simulink model "Compression_Gain_Calc"  (R2019a)
settings: Solver=FixedStepDiscrete  StartTime=0.0  StopTime=t_end  RelTol=1e-3
InitFcn:
  | clear;
  | DIAGNOSTIC = 0;  %% flag to give more information as simulation proceeds such as comments & plots
  | CALIB_DIAGNOSTIC =  0; %% flag to give more information about calibration of filterbank due to overlap between filters: Mar 2016
  | PRESCRIPT = 1;  %% flag to plot requested versus achieved insertion gains (esp for 125-250 Hz region).
  | ipfiledigrms = -36; %% input file RMS in dB for 65 dB SPL equivalent
  | opfiledigrms = -36; %% output file RMS in dB for 65 dB SPL equivalent
  | equiv_ipSPL = 65; %% simulation of signal at this level through aid`
  | X_high = 1; % Maximum input
  | ref_dB = 85; X_ref = 1; % Define a reference point in X and its dBA value
  | re_level = 10.^(.05*(equiv_ipSPL-65)); %% scale factor at start of hearing aid, to get input to desired simulation level
  | M_bits = 5;   % decides length of tables, 2^(4+M_bits)
  | 
  | NChans = 5;
  | [chan_cfs, chan_thrs, t_atts, t_rels] ...
  |    = InitializeCompressionSettings(NChans);
  | % AidSettings5Chans;
  | 
  | %[VALID_WAV_FILE, sig, Fs, nbits, file_rms_dB, NStreams] ...
  | %  = loadwavfile(ipfiledigrms); %%  find [Fs], performs [recalculate] externally, provided valid file found
  | VALID_WAV_FILE = 1;
  | %[newfile, newpath] = uigetfile('*.wav','Open Signal File To Process.....');
  | %if isequal(newfile,0) || isequal(newpath,0)
  | %    fprintf(1,'\nFile not found'); VALID_WAV_FILE = 0;
  | %else
  | %    [sig, Fs] = audioread(strcat(newpath,newfile));
  | %end
  | X_thresh = 1*10^(0.05*(0-85));
  | 
  | Amplitudes = [X_thresh, X_thresh*10, X_thresh*100, X_thresh*1000, X_thresh*10000, 1]; %, X_thresh*100000];
  | 
  | fMin = 100; %Hz
  | fMax = 10000; %Hz
  | Fs = 48000; %Hz
  | Ts = 1/Fs;
  | %tt = (0:length(sig)-1 )./Fs;
  | tt = 0:Ts:4;
  | deltaF = (fMax - fMin)/tt(end);
  | X_sweep = Amplitudes'*sin(2*pi*(fMin*tt +  0.5*deltaF*tt.*tt)) ;
  | 
  | Fs = 48000;
  | Volume = 6;
  | sig = X_sweep(Volume,:)';
  | opplayer  = audioplayer(sig, Fs);
  | nbits = opplayer.bitspersample;
  | %sig = resample(sig,48000,Fs);
  | %Fs = 48000;
  | 
  | 
  | NStreams = min(size(sig));
  | EQ_SPAN_MSEC = 6;
  | 
  | insrt_frqs = [125, 250, 500, 1000, 2000, 3000, 4000, 6000, 8000, 10000 ]; %% decimal values
  | insrt_gns = [0 3 5 10 15 20 25 30 30 30]; %% prescribed dB for 65 dB input
  | %insrt_gns = 5*ones(1,length(insrt_frqs));  %no prescription
  | n_insrts = length(insrt_gns);
  | 
  | UPPER_FREQ_LIM = min(11e3, 0.90*Fs/2);
  | [ig_eq, calib_bpfs, dig_chan_lvl_0dBgain, dig_chan_dBthrs, Calib_recomb_dBpost] ...
  |     = update_channel_params(Fs, NChans, chan_cfs, chan_thrs, insrt_frqs, insrt_gns, ...
  |     0.1, UPPER_FREQ_LIM, EQ_SPAN_MSEC, PRESCRIPT, DIAGNOSTIC, CALIB_DIAGNOSTIC) ;  %% calculates channel edge frequencies, generates expected band levels for LTASS SWN to calibrate compressors & filterbank
  | 
  | recombGain = 10.^(0.05.*Calib_recomb_dBpost);
  | 
  | % translate sig into a form simulink likes
  | % Ts = 1/Fs;
  | % tt = (0:length(sig)-1).*Ts;
  | %t_end = tt(5*2^(M_bits+4) );   % to test table fill
  | t_end = tt(end);
  | sig_in = [tt', sig];
  | min_thresh_dB = 0;
  | for ix = 1:NChans
  |    [Gain_Table(:,ix), max_gain_prescript(ix), X_in(:,ix), chan_crs(ix)] ...
  |      = Compression_Wrapper_V2(Fs, min_thresh_dB, ...
  |      X_high, calib_bpfs(:,ix), ig_eq, ref_dB, X_ref, M_bits);
  | end
  | 
  | Initialize_Delay_Values;
  | Initialize_AGC_Consts;
  | W_bits = 32;
  | F_bits = 28;
  | M_bits = 5;
  | M_Bits = M_bits;
  | 
  | % Generating signals for simulink
  | Table_Fill = zeros(1,length(tt))';
  | Table_Fill(1                : 2^(M_bits+4) )  = Gain_Table(:,1);
  | Table_Fill(2^(M_bits+4)+1   : 2*2^(M_bits+4) )= Gain_Table(:,2);
  | Table_Fill(2*2^(M_bits+4)+1 : 3*2^(M_bits+4) )= Gain_Table(:,3);
  | Table_Fill(3*2^(M_bits+4)+1 : 4*2^(M_bits+4) )= Gain_Table(:,4);
  | Table_Fill(4*2^(M_bits+4)+1 : 5*2^(M_bits+4) )= Gain_Table(:,5);
  | Table_Fill_t = [tt', Table_Fill];
  | Fill_Valid = zeros(1,length(tt))';
  | Fill_Valid(1:5*2^(M_bits+4)) = 1;
  | Fill_Valid = boolean(Fill_Valid);
  | Fill_Valid_t = [tt', Fill_Valid];
  | t_att = t_atts./1000; s_att = t_att.*Fs; % change units of t_atts from ms to samples
  | t_rel = t_rels./1000; s_rel = t_rel.*Fs; % change units of t_rels from ms to samples
  | r_att = nthroot(0.1, s_att);
  | r_rel = nthroot(0.1, s_rel);
  | 
  | Reset = [tt', boolean(zeros(1,length(tt)))'];
StopFcn:
  | proc_sig = double(out.proc_sig.data(:));
  | %alignedSigs = double(out.alignedSigs.data(:));
  | [opwav, stop_ok] = savewavfile(opfiledigrms, ipfiledigrms, proc_sig, Fs, nbits, NStreams);
  | 
  | load('SweepSimOutput.mat')
  | X_out_Sweep_Sim(Volume,:) = proc_sig;
  | save('SweepSimOutput.mat', 'X_out_Sweep_Sim');
undefined symbols (not defined in the file or in its folder): Ts_system
libraries: simulink x68, hdlsllib x51
(part 1 of 2)
settings Model: Creator=Bailey  LastModifiedBy=Bailey
settings DataIOCC: InitialState=Table_Fill(1: 2^(M_bits+4) )  SaveOutput=off  SaveTime=off
settings OptimizationCC: BlockReduction=off  ConditionallyExecuteInputs=off  DefaultParameterBehavior=Inlined
settings DebuggingCC: AlgebraicLoopMsg=error  SingleTaskRateTransMsg=error
settings HardwareCC: ProdBitPerPointer=32  ProdBitPerSizeT=32  ProdBitPerPtrDiffT=32  ProdLargestAtomicFloat=None  ProdIntDivRoundTo=Undefined  ProdEndianess=Unspecified  ProdWordSize=32  ProdHWDeviceType=ASIC/FPGA->ASIC/FPGA  TargetBitPerPointer=64  TargetBitPerSizeT=64  TargetBitPerPtrDiffT=64  TargetLongLongMode=on  TargetIntDivRoundTo=Zero  TargetEndianess=LittleEndian  TargetWordSize=64  TargetHWDeviceType=Custom Processor->MATLAB Host Computer  ProdEqTarget=off

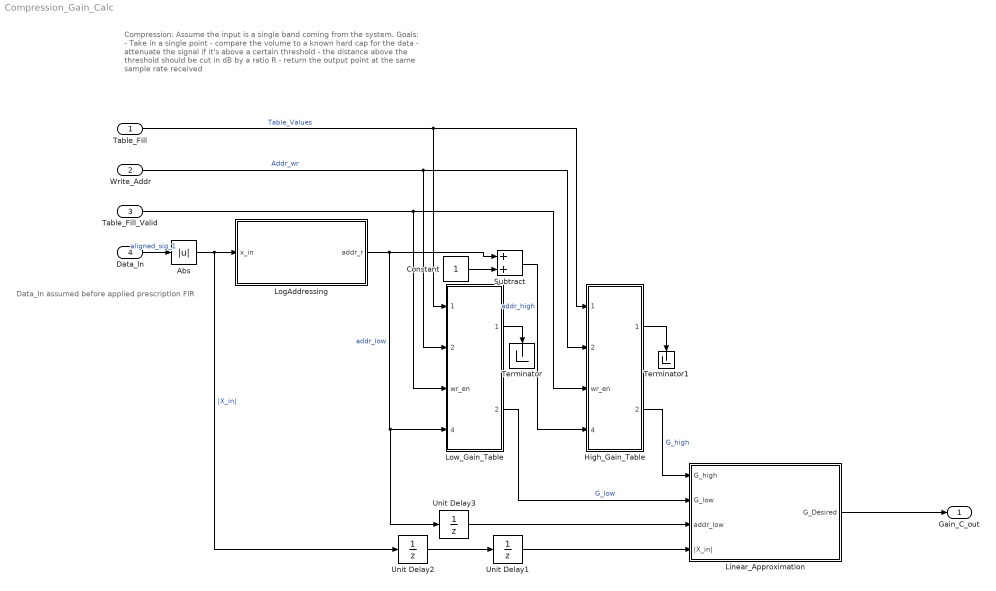
== system Compression_Gain_Calc ==
  note: Data_In assumed before applied prescription FIR
  note: Compression: Assume the input is a single band coming from the system.
      |
      | Goals:
      | 	- Take in a single point
      | 	- compare the volume to a known hard cap for the data
      | 	- attenuate the signal if it's above a certain threshold
      | 		- the distance above the threshold should be cut in dB by a ratio R
      | 	- return the output point at the same sample rate received
  Table_Fill : Inport  OutDataTypeStr=fixdt(1,32,28)  PortDimensions=1  SampleTime=[2.0833333333333333e-05,0]
  Write_Addr : Inport  Port=2  OutDataTypeStr=fixdt(0,9,0)  PortDimensions=1  SampleTime=[2.0833333333333333e-05,0]
  Table_Fill_Valid : Inport  Port=3  OutDataTypeStr=boolean  PortDimensions=1  SampleTime=[2.0833333333333333e-05,0]
  Data_In : Inport  Port=4  OutDataTypeStr=fixdt(1,32,28)  PortDimensions=1  SampleTime=[2.0833333333333333e-05,0]
  Abs : Abs
  Constant : Constant  OutDataTypeStr=fixdt(0,9,0)  SampleTime=-1
  High_Gain_Table : Subsystem  AncestorBlock=hdlsllibUNLOCKED/HDL RAMs/Dual Port RAM  mask(Dual-port RAM){ram_size=4+M_Bits}
      mask prompts: ram_size "Address port width (2 to 29 bits)"
      mask help: This block simulates a dual-port RAM with two data output ports.
      mask init:
      | hdlblkmask_dpram;
      mask Help: helpview([docroot '/simulink/helptargets.map'],'HDL_dual_port_RAM');
  Linear_Approximation : Subsystem
  LogAddressing : Subsystem
  Low_Gain_Table : Subsystem  AncestorBlock=hdlsllibUNLOCKED/HDL RAMs/Dual Port RAM  mask(Dual-port RAM){ram_size=4+M_Bits}
      mask prompts: ram_size "Address port width (2 to 29 bits)"
      mask help: This block simulates a dual-port RAM with two data output ports.
      mask init:
      | hdlblkmask_dpram;
      mask Help: helpview([docroot '/simulink/helptargets.map'],'HDL_dual_port_RAM');
  Subtract : Sum  OutDataTypeStr=Inherit: Same as first input
  Terminator : Terminator
  Terminator1 : Terminator
  Unit Delay1 : UnitDelay  InitialCondition=1  SampleTime=-1  HasFrameUpgradeWarning=on
  Unit Delay2 : UnitDelay  InitialCondition=1  SampleTime=-1  HasFrameUpgradeWarning=on
  Unit Delay3 : UnitDelay  InitialCondition=1  SampleTime=-1  HasFrameUpgradeWarning=on
  Gain_C_out : Outport  OutDataTypeStr=fixdt(1,32,28)  PortDimensions=1  SampleTime=[2.0833333333333333e-05,0]
  wires:
  Table_Fill/1 -> Low_Gain_Table/1(wr_din), High_Gain_Table/1(wr_din)  "Table_Values"
  Table_Fill_Valid/1 -> Low_Gain_Table/3(wr_en), High_Gain_Table/3(wr_en)
  Write_Addr/1 -> Low_Gain_Table/2(wr_addr), High_Gain_Table/2(wr_addr)  "Addr_wr"
  LogAddressing/1(addr_r) -> Subtract/1, Unit Delay3/1, Low_Gain_Table/4(rd_addr)  "addr_low"
  Abs/1 -> LogAddressing/1(x_in), Unit Delay2/1  "|X_in|"
  Data_In/1 -> Abs/1  "aligned_sig_1"
  Constant/1 -> Subtract/2
  Subtract/1 -> High_Gain_Table/4(rd_addr)  "addr_high"
  Low_Gain_Table/1(wr_dout) -> Terminator/1
  High_Gain_Table/1(wr_dout) -> Terminator1/1
  High_Gain_Table/2(rd_dout) -> Linear_Approximation/1(G_high)  "G_high"
  Low_Gain_Table/2(rd_dout) -> Linear_Approximation/2(G_low)  "G_low"
  Linear_Approximation/1(G_Desired) -> Gain_C_out/1
  Unit Delay2/1 -> Unit Delay1/1
  Unit Delay1/1 -> Linear_Approximation/4(|X_in|)
  Unit Delay3/1 -> Linear_Approximation/3(addr_low)

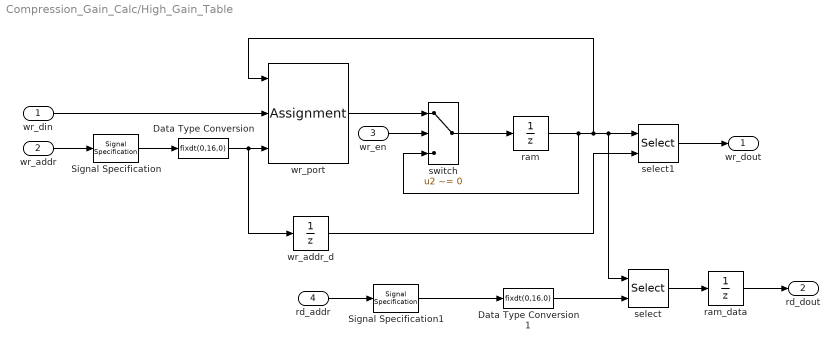
== system Compression_Gain_Calc/High_Gain_Table ==
  wr_din : Inport
  wr_addr : Inport  Port=2
  wr_en : Inport  Port=3  OutDataTypeStr=boolean
  rd_addr : Inport  Port=4
  Data Type Conversion : DataTypeConversion  OutDataTypeStr=fixdt(0,16,0)
  Data Type Conversion1 : DataTypeConversion  OutDataTypeStr=fixdt(0,16,0)
  Signal Specification : SignalSpecification  OutDataTypeStr=fixdt(0,ram_size,0)  Dimensions=1
  Signal Specification1 : SignalSpecification  OutDataTypeStr=fixdt(0,ram_size,0)  Dimensions=1
  ram : UnitDelay  InitialCondition=Table_Fill_t(2^(M_bits+4) +1 : 2*2^(M_bits+4) )  SampleTime=-1  HasFrameUpgradeWarning=on
  ram_data : UnitDelay  SampleTime=-1  HasFrameUpgradeWarning=on
  select : Selector  IndexMode=Zero-based  InputPortWidth=2^ram_size  IndexOptions=Index vector (port)  Indices=[1 3]  OutputSizes=1
  select1 : Selector  IndexMode=Zero-based  InputPortWidth=2^ram_size  IndexOptions=Index vector (port)  Indices=[1 3]  OutputSizes=1
  switch : Switch  Criteria=u2 ~= 0
  wr_addr_d : UnitDelay  SampleTime=-1  HasFrameUpgradeWarning=on
  wr_port : Assignment  IndexMode=Zero-based  IndexOptions=Index vector (port)  Indices=1  OutputSizes=[1 1]
  wr_dout : Outport
  rd_dout : Outport  Port=2
  wires:
  Data Type Conversion1/1 -> select/2
  Data Type Conversion/1 -> wr_addr_d/1, wr_port/3
  wr_addr_d/1 -> select1/2
  select1/1 -> wr_dout/1
  Signal Specification1/1 -> Data Type Conversion1/1
  Signal Specification/1 -> Data Type Conversion/1
  select/1 -> ram_data/1
  rd_addr/1 -> Signal Specification1/1
  wr_en/1 -> switch/2
  wr_din/1 -> wr_port/2
  ram/1 -> switch/3, select1/1, select/1, wr_port/1
  switch/1 -> ram/1
  wr_port/1 -> switch/1
  wr_addr/1 -> Signal Specification/1
  ram_data/1 -> rd_dout/1

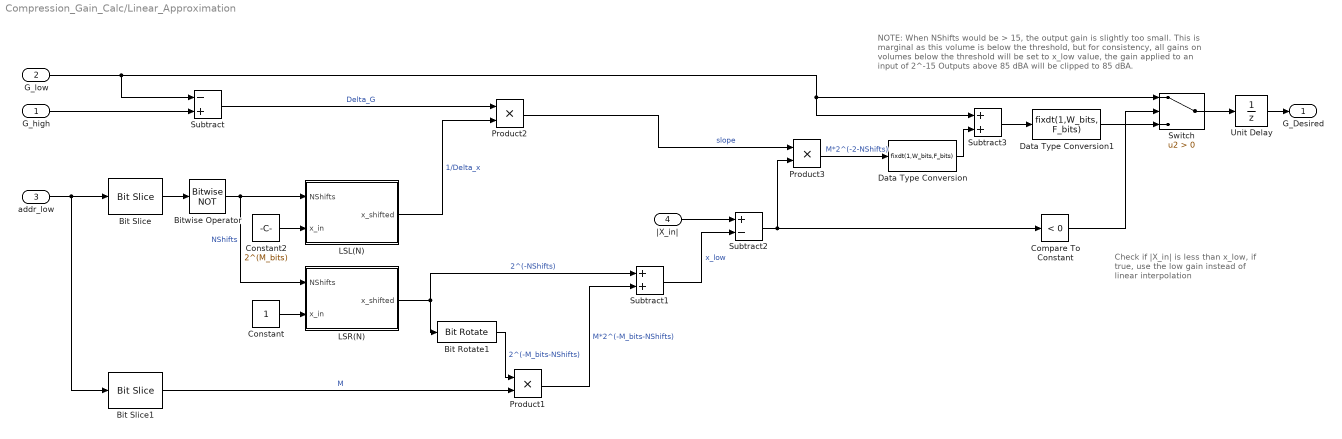
== system Compression_Gain_Calc/Linear_Approximation ==
  note: NOTE: When NShifts would be > 15, the output gain is slightly too small.
      | This is marginal as this volume is below the threshold, but for consistency,
      | all gains on volumes below the threshold will be set to x_low value, the
      | gain applied to an input of 2^-15
      | Outputs above 85 dBA will be clipped to 85 dBA.
  note: Check if |X_in| is less than x_low,
      | if true, use the low gain instead of
      | linear interpolation
  G_high : Inport
  G_low : Inport  Port=2
  addr_low : Inport  Port=3
  |X_in| : Inport  Port=4
  Bit Rotate1 : hdlsllib/Logic and Bit Operations/Bit Rotate  mode=Rotate Right  N=M_Bits
      settings: SourceProductName=Simulink  SourceProductBaseCode=SL
  Bit Slice : hdlsllib/Logic and Bit Operations/Bit Slice  lidx=M_Bits+3  ridx=M_Bits
      settings: SourceProductName=Simulink  SourceProductBaseCode=SL
  Bit Slice1 : hdlsllib/Logic and Bit Operations/Bit Slice  lidx=M_Bits-1  ridx=0
      settings: SourceProductName=Simulink  SourceProductBaseCode=SL
  Bitwise Operator : simulink/Logic and Bit Operations/Bitwise Operator  logicop=NOT  UseBitMask=off  BitMask=bin2dec('11011001')  BitMaskRealWorld=Stored Integer
  Compare To Constant : simulink/Logic and Bit Operations/Compare To Constant  relop=<  const=0  OutDataTypeStr=boolean
  Constant : Constant  OutDataTypeStr=fixdt(0,W_bits,W_bits-2)  SampleTime=-1
  Constant2 : Constant  Value=2^(M_bits)  OutDataTypeStr=fixdt(0,W_bits,0)  SampleTime=-1
  Data Type Conversion : DataTypeConversion  OutDataTypeStr=fixdt(1,W_bits,F_bits)
  Data Type Conversion1 : DataTypeConversion  OutDataTypeStr=fixdt(1,W_bits, F_bits)
  LSL(N) : Subsystem
  LSR(N) : Subsystem
  Product1 : Product
  Product2 : Product
  Product3 : Product
  Subtract : Sum  Inputs=-+
  Subtract1 : Sum  OutDataTypeStr=fixdt(1,W_bits, F_bits)
  Subtract2 : Sum  Inputs=+-  OutDataTypeStr=Inherit: Same as first input
  Subtract3 : Sum
  Switch : Switch  Criteria=u2 > Threshold
  Unit Delay : UnitDelay  InitialCondition=1  SampleTime=-1  HasFrameUpgradeWarning=on
  G_Desired : Outport
  wires:
  Switch/1 -> Unit Delay/1
  Compare To Constant/1 -> Switch/2
  Unit Delay/1 -> G_Desired/1
  Data Type Conversion1/1 -> Switch/3
  Data Type Conversion/1 -> Subtract3/2
  Constant2/1 -> LSL(N)/2(x_in)
  Subtract3/1 -> Data Type Conversion1/1
  Product3/1 -> Data Type Conversion/1  "M*2^(-2-NShifts)"
  Subtract2/1 -> Product3/2, Compare To Constant/1
  |X_in|/1 -> Subtract2/1
  Product2/1 -> Product3/1  "slope"
  LSL(N)/1(x_shifted) -> Product2/2  "1/Delta_x"
  Subtract1/1 -> Subtract2/2  "x_low"
  Product1/1 -> Subtract1/2  "M*2^(-M_bits-NShifts)"
  Bit Rotate1/1 -> Product1/1  "2^(-M_bits-NShifts)"
  LSR(N)/1(x_shifted) -> Subtract1/1, Bit Rotate1/1  "2^(-NShifts)"
  Constant/1 -> LSR(N)/2(x_in)
  Subtract/1 -> Product2/1  "Delta_G"
  G_low/1 -> Subtract3/1, Switch/1, Subtract/1
  G_high/1 -> Subtract/2
  Bit Slice1/1 -> Product1/2  "M"
  Bitwise Operator/1 -> LSL(N)/1(NShifts), LSR(N)/1(NShifts)  "NShifts"
  Bit Slice/1 -> Bitwise Operator/1
  addr_low/1 -> Bit Slice/1, Bit Slice1/1

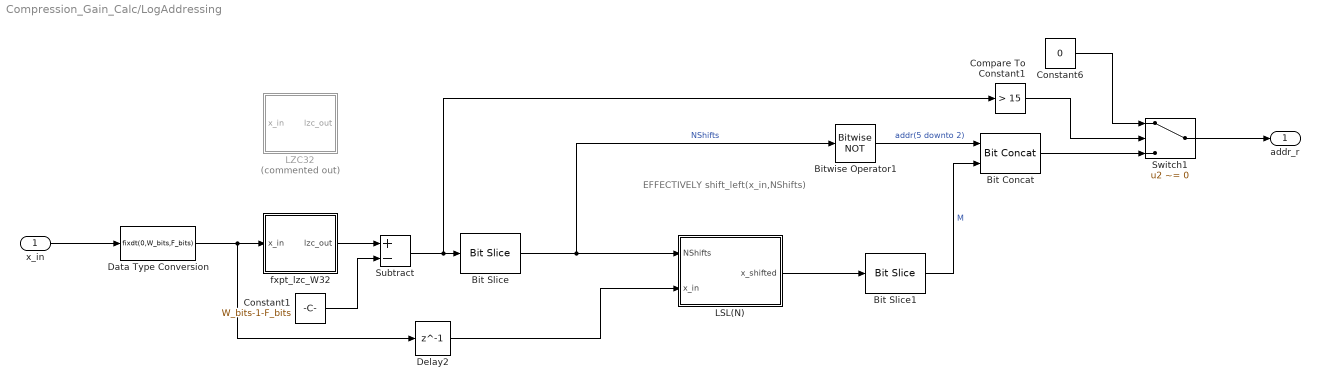
== system Compression_Gain_Calc/LogAddressing ==
  note: EFFECTIVELY shift_left(x_in,NShifts)
  x_in : Inport
  Bit Concat : hdlsllib/Logic and Bit Operations/Bit Concat  numInputs=2
      settings: SourceProductName=Simulink
  Bit Slice : hdlsllib/Logic and Bit Operations/Bit Slice  lidx=3  ridx=0
      settings: SourceProductName=Simulink  SourceProductBaseCode=SL
  Bit Slice1 : hdlsllib/Logic and Bit Operations/Bit Slice  lidx=F_bits-1  ridx=F_bits-M_bits
      settings: SourceProductName=Simulink  SourceProductBaseCode=SL
  Bitwise Operator1 : simulink/Logic and Bit Operations/Bitwise Operator  logicop=NOT  UseBitMask=off  BitMask=bin2dec('11011001')  BitMaskRealWorld=Stored Integer
  Compare To Constant1 : simulink/Logic and Bit Operations/Compare To Constant  relop=>  const=15  OutDataTypeStr=boolean
  Constant1 : Constant  Value=W_bits-1-F_bits  OutDataTypeStr=fixdt(0,6,0)  SampleTime=-1
  Constant6 : Constant  Value=0  OutDataTypeStr=fixdt(0,9,0)  SampleTime=-1
  Data Type Conversion : DataTypeConversion  OutDataTypeStr=fixdt(0,W_bits,F_bits)
  Delay2 : Delay  DelayLength=1  SampleTime=Ts_system
  LSL(N) : Subsystem
  LZC32 : Subsystem  Commented=on  TreatAsAtomicUnit=on
  Subtract : Sum  Inputs=+-  OutDataTypeStr=Inherit: Same as first input
  Switch1 : Switch  Criteria=u2 ~= 0
  fxpt_lzc_W32 : Subsystem  TreatAsAtomicUnit=on
  addr_r : Outport
  wires:
  Subtract/1 -> Bit Slice/1, Compare To Constant1/1
  Compare To Constant1/1 -> Switch1/2
  Switch1/1 -> addr_r/1
  Constant6/1 -> Switch1/1
  Data Type Conversion/1 -> Delay2/1, fxpt_lzc_W32/1(x_in)
  LSL(N)/1(x_shifted) -> Bit Slice1/1
  Delay2/1 -> LSL(N)/2(x_in)
  Bit Slice/1 -> LSL(N)/1(NShifts), Bitwise Operator1/1  "NShifts"
  Constant1/1 -> Subtract/2
  Bit Concat/1 -> Switch1/3
  fxpt_lzc_W32/1(lzc_out) -> Subtract/1
  Bitwise Operator1/1 -> Bit Concat/1  "addr(5 downto 2)"
  Bit Slice1/1 -> Bit Concat/2  "M"
  x_in/1 -> Data Type Conversion/1

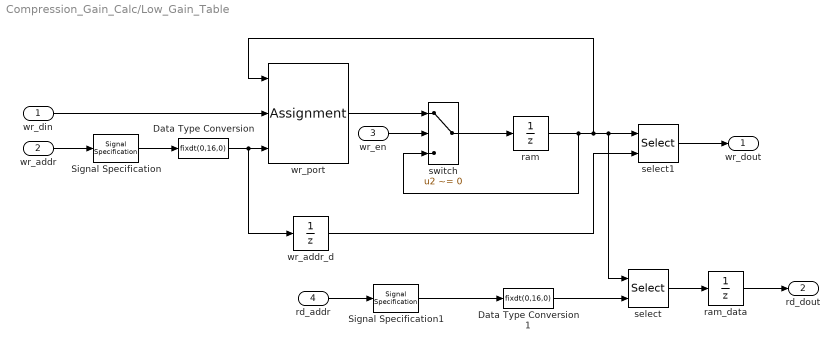
== system Compression_Gain_Calc/Low_Gain_Table ==
  wr_din : Inport
  wr_addr : Inport  Port=2
  wr_en : Inport  Port=3  OutDataTypeStr=boolean
  rd_addr : Inport  Port=4
  Data Type Conversion : DataTypeConversion  OutDataTypeStr=fixdt(0,16,0)
  Data Type Conversion1 : DataTypeConversion  OutDataTypeStr=fixdt(0,16,0)
  Signal Specification : SignalSpecification  OutDataTypeStr=fixdt(0,ram_size,0)  Dimensions=1
  Signal Specification1 : SignalSpecification  OutDataTypeStr=fixdt(0,ram_size,0)  Dimensions=1
  ram : UnitDelay  InitialCondition=Table_Fill_t(1: 2^(M_bits+4) )  SampleTime=-1  HasFrameUpgradeWarning=on
  ram_data : UnitDelay  SampleTime=-1  HasFrameUpgradeWarning=on
  select : Selector  IndexMode=Zero-based  InputPortWidth=2^ram_size  IndexOptions=Index vector (port)  Indices=[1 3]  OutputSizes=1
  select1 : Selector  IndexMode=Zero-based  InputPortWidth=2^ram_size  IndexOptions=Index vector (port)  Indices=[1 3]  OutputSizes=1
  switch : Switch  Criteria=u2 ~= 0
  wr_addr_d : UnitDelay  SampleTime=-1  HasFrameUpgradeWarning=on
  wr_port : Assignment  IndexMode=Zero-based  IndexOptions=Index vector (port)  Indices=1  OutputSizes=[1 1]
  wr_dout : Outport
  rd_dout : Outport  Port=2
  wires:
  Data Type Conversion1/1 -> select/2
  Data Type Conversion/1 -> wr_addr_d/1, wr_port/3
  wr_addr_d/1 -> select1/2
  select1/1 -> wr_dout/1
  Signal Specification1/1 -> Data Type Conversion1/1
  Signal Specification/1 -> Data Type Conversion/1
  select/1 -> ram_data/1
  rd_addr/1 -> Signal Specification1/1
  wr_en/1 -> switch/2
  wr_din/1 -> wr_port/2
  ram/1 -> switch/3, select1/1, select/1, wr_port/1
  switch/1 -> ram/1
  wr_port/1 -> switch/1
  wr_addr/1 -> Signal Specification/1
  ram_data/1 -> rd_dout/1

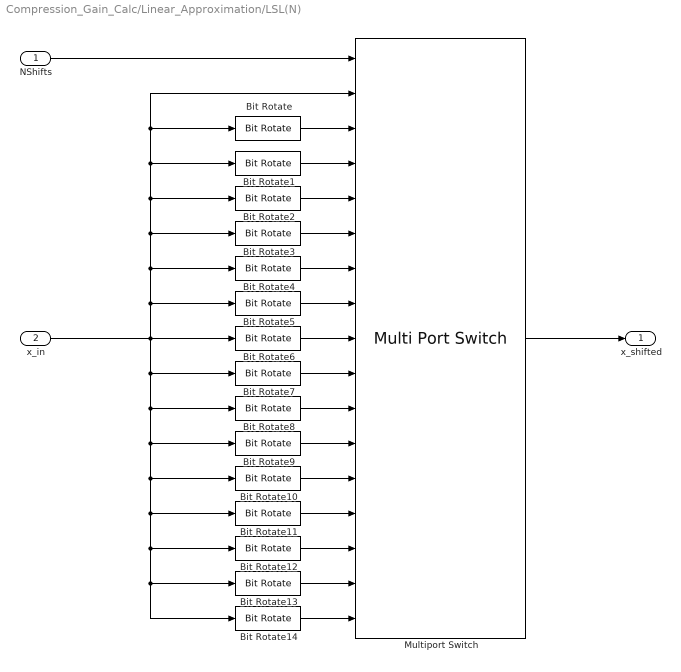
== system Compression_Gain_Calc/Linear_Approximation/LSL(N) ==
  NShifts : Inport
  x_in : Inport  Port=2
  Bit Rotate : hdlsllib/Logic and Bit Operations/Bit Rotate  mode=Rotate Left  N=1
      settings: SourceProductName=Simulink  SourceProductBaseCode=SL
  Bit Rotate1 : hdlsllib/Logic and Bit Operations/Bit Rotate  mode=Rotate Left  N=2
      settings: SourceProductName=Simulink  SourceProductBaseCode=SL
  Bit Rotate10 : hdlsllib/Logic and Bit Operations/Bit Rotate  mode=Rotate Left  N=11
      settings: SourceProductName=Simulink  SourceProductBaseCode=SL
  Bit Rotate11 : hdlsllib/Logic and Bit Operations/Bit Rotate  mode=Rotate Left  N=12
      settings: SourceProductName=Simulink  SourceProductBaseCode=SL
  Bit Rotate12 : hdlsllib/Logic and Bit Operations/Bit Rotate  mode=Rotate Left  N=13
      settings: SourceProductName=Simulink  SourceProductBaseCode=SL
  Bit Rotate13 : hdlsllib/Logic and Bit Operations/Bit Rotate  mode=Rotate Left  N=14
      settings: SourceProductName=Simulink  SourceProductBaseCode=SL
  Bit Rotate14 : hdlsllib/Logic and Bit Operations/Bit Rotate  mode=Rotate Left  N=15
      settings: SourceProductName=Simulink  SourceProductBaseCode=SL
  Bit Rotate2 : hdlsllib/Logic and Bit Operations/Bit Rotate  mode=Rotate Left  N=3
      settings: SourceProductName=Simulink  SourceProductBaseCode=SL
  Bit Rotate3 : hdlsllib/Logic and Bit Operations/Bit Rotate  mode=Rotate Left  N=4
      settings: SourceProductName=Simulink  SourceProductBaseCode=SL
  Bit Rotate4 : hdlsllib/Logic and Bit Operations/Bit Rotate  mode=Rotate Left  N=5
      settings: SourceProductName=Simulink  SourceProductBaseCode=SL
  Bit Rotate5 : hdlsllib/Logic and Bit Operations/Bit Rotate  mode=Rotate Left  N=6
      settings: SourceProductName=Simulink  SourceProductBaseCode=SL
  Bit Rotate6 : hdlsllib/Logic and Bit Operations/Bit Rotate  mode=Rotate Left  N=7
      settings: SourceProductName=Simulink  SourceProductBaseCode=SL
  Bit Rotate7 : hdlsllib/Logic and Bit Operations/Bit Rotate  mode=Rotate Left  N=8
      settings: SourceProductName=Simulink  SourceProductBaseCode=SL
  Bit Rotate8 : hdlsllib/Logic and Bit Operations/Bit Rotate  mode=Rotate Left  N=9
      settings: SourceProductName=Simulink  SourceProductBaseCode=SL
  Bit Rotate9 : hdlsllib/Logic and Bit Operations/Bit Rotate  mode=Rotate Left  N=10
      settings: SourceProductName=Simulink  SourceProductBaseCode=SL
  Multiport Switch : MultiPortSwitch  DataPortOrder=Zero-based contiguous  Inputs=16  DiagnosticForDefault=Warning  zeroidx=on
  x_shifted : Outport
  wires:
  Bit Rotate14/1 -> Multiport Switch/17
  Bit Rotate13/1 -> Multiport Switch/16
  Bit Rotate12/1 -> Multiport Switch/15
  Bit Rotate11/1 -> Multiport Switch/14
  Bit Rotate10/1 -> Multiport Switch/13
  Bit Rotate9/1 -> Multiport Switch/12
  Bit Rotate8/1 -> Multiport Switch/11
  Bit Rotate7/1 -> Multiport Switch/10
  Bit Rotate6/1 -> Multiport Switch/9
  Bit Rotate5/1 -> Multiport Switch/8
  Bit Rotate4/1 -> Multiport Switch/7
  Bit Rotate3/1 -> Multiport Switch/6
  Bit Rotate2/1 -> Multiport Switch/5
  Bit Rotate1/1 -> Multiport Switch/4
  Bit Rotate/1 -> Multiport Switch/3
  x_in/1 -> Bit Rotate6/1, Bit Rotate3/1, Bit Rotate2/1, Bit Rotate1/1, Bit Rotate/1, Multiport Switch/2, Bit Rotate4/1, Bit Rotate5/1, Bit Rotate7/1, Bit Rotate8/1, Bit Rotate9/1, Bit Rotate10/1, Bit Rotate11/1, Bit Rotate14/1, Bit Rotate13/1, Bit Rotate12/1
  Multiport Switch/1 -> x_shifted/1
  NShifts/1 -> Multiport Switch/1

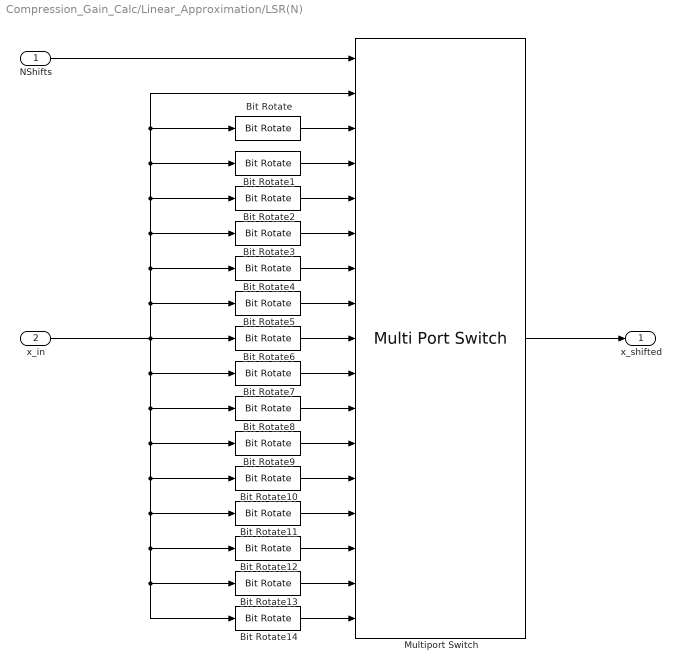
== system Compression_Gain_Calc/Linear_Approximation/LSR(N) ==
  NShifts : Inport
  x_in : Inport  Port=2
  Bit Rotate : hdlsllib/Logic and Bit Operations/Bit Rotate  mode=Rotate Right  N=1
      settings: SourceProductName=Simulink  SourceProductBaseCode=SL
  Bit Rotate1 : hdlsllib/Logic and Bit Operations/Bit Rotate  mode=Rotate Right  N=2
      settings: SourceProductName=Simulink  SourceProductBaseCode=SL
  Bit Rotate10 : hdlsllib/Logic and Bit Operations/Bit Rotate  mode=Rotate Right  N=11
      settings: SourceProductName=Simulink  SourceProductBaseCode=SL
  Bit Rotate11 : hdlsllib/Logic and Bit Operations/Bit Rotate  mode=Rotate Right  N=12
      settings: SourceProductName=Simulink  SourceProductBaseCode=SL
  Bit Rotate12 : hdlsllib/Logic and Bit Operations/Bit Rotate  mode=Rotate Right  N=13
      settings: SourceProductName=Simulink  SourceProductBaseCode=SL
  Bit Rotate13 : hdlsllib/Logic and Bit Operations/Bit Rotate  mode=Rotate Right  N=14
      settings: SourceProductName=Simulink  SourceProductBaseCode=SL
  Bit Rotate14 : hdlsllib/Logic and Bit Operations/Bit Rotate  mode=Rotate Right  N=15
      settings: SourceProductName=Simulink  SourceProductBaseCode=SL
  Bit Rotate2 : hdlsllib/Logic and Bit Operations/Bit Rotate  mode=Rotate Right  N=3
      settings: SourceProductName=Simulink  SourceProductBaseCode=SL
  Bit Rotate3 : hdlsllib/Logic and Bit Operations/Bit Rotate  mode=Rotate Right  N=4
      settings: SourceProductName=Simulink  SourceProductBaseCode=SL
  Bit Rotate4 : hdlsllib/Logic and Bit Operations/Bit Rotate  mode=Rotate Right  N=5
      settings: SourceProductName=Simulink  SourceProductBaseCode=SL
  Bit Rotate5 : hdlsllib/Logic and Bit Operations/Bit Rotate  mode=Rotate Right  N=6
      settings: SourceProductName=Simulink  SourceProductBaseCode=SL
  Bit Rotate6 : hdlsllib/Logic and Bit Operations/Bit Rotate  mode=Rotate Right  N=7
      settings: SourceProductName=Simulink  SourceProductBaseCode=SL
  Bit Rotate7 : hdlsllib/Logic and Bit Operations/Bit Rotate  mode=Rotate Right  N=8
      settings: SourceProductName=Simulink  SourceProductBaseCode=SL
  Bit Rotate8 : hdlsllib/Logic and Bit Operations/Bit Rotate  mode=Rotate Right  N=9
      settings: SourceProductName=Simulink  SourceProductBaseCode=SL
  Bit Rotate9 : hdlsllib/Logic and Bit Operations/Bit Rotate  mode=Rotate Right  N=10
      settings: SourceProductName=Simulink  SourceProductBaseCode=SL
  Multiport Switch : MultiPortSwitch  DataPortOrder=Zero-based contiguous  Inputs=16  DiagnosticForDefault=Warning  zeroidx=on
  x_shifted : Outport
  wires:
  Bit Rotate14/1 -> Multiport Switch/17
  Bit Rotate13/1 -> Multiport Switch/16
  Bit Rotate12/1 -> Multiport Switch/15
  Bit Rotate11/1 -> Multiport Switch/14
  Bit Rotate10/1 -> Multiport Switch/13
  Bit Rotate9/1 -> Multiport Switch/12
  Bit Rotate8/1 -> Multiport Switch/11
  Bit Rotate7/1 -> Multiport Switch/10
  Bit Rotate6/1 -> Multiport Switch/9
  Bit Rotate5/1 -> Multiport Switch/8
  Bit Rotate4/1 -> Multiport Switch/7
  Bit Rotate3/1 -> Multiport Switch/6
  Bit Rotate2/1 -> Multiport Switch/5
  Bit Rotate1/1 -> Multiport Switch/4
  Bit Rotate/1 -> Multiport Switch/3
  x_in/1 -> Bit Rotate6/1, Bit Rotate3/1, Bit Rotate2/1, Bit Rotate1/1, Bit Rotate/1, Multiport Switch/2, Bit Rotate4/1, Bit Rotate5/1, Bit Rotate7/1, Bit Rotate8/1, Bit Rotate9/1, Bit Rotate10/1, Bit Rotate11/1, Bit Rotate14/1, Bit Rotate13/1, Bit Rotate12/1
  Multiport Switch/1 -> x_shifted/1
  NShifts/1 -> Multiport Switch/1

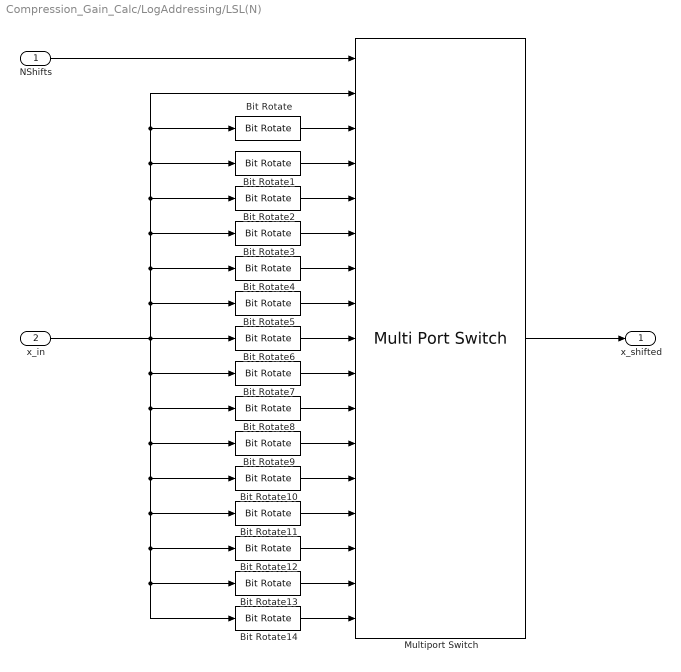
== system Compression_Gain_Calc/LogAddressing/LSL(N) ==
  NShifts : Inport
  x_in : Inport  Port=2
  Bit Rotate : hdlsllib/Logic and Bit Operations/Bit Rotate  mode=Rotate Left  N=1
      settings: SourceProductName=Simulink  SourceProductBaseCode=SL
  Bit Rotate1 : hdlsllib/Logic and Bit Operations/Bit Rotate  mode=Rotate Left  N=2
      settings: SourceProductName=Simulink  SourceProductBaseCode=SL
  Bit Rotate10 : hdlsllib/Logic and Bit Operations/Bit Rotate  mode=Rotate Left  N=11
      settings: SourceProductName=Simulink  SourceProductBaseCode=SL
  Bit Rotate11 : hdlsllib/Logic and Bit Operations/Bit Rotate  mode=Rotate Left  N=12
      settings: SourceProductName=Simulink  SourceProductBaseCode=SL
  Bit Rotate12 : hdlsllib/Logic and Bit Operations/Bit Rotate  mode=Rotate Left  N=13
      settings: SourceProductName=Simulink  SourceProductBaseCode=SL
  Bit Rotate13 : hdlsllib/Logic and Bit Operations/Bit Rotate  mode=Rotate Left  N=14
      settings: SourceProductName=Simulink  SourceProductBaseCode=SL
  Bit Rotate14 : hdlsllib/Logic and Bit Operations/Bit Rotate  mode=Rotate Left  N=15
      settings: SourceProductName=Simulink  SourceProductBaseCode=SL
  Bit Rotate2 : hdlsllib/Logic and Bit Operations/Bit Rotate  mode=Rotate Left  N=3
      settings: SourceProductName=Simulink  SourceProductBaseCode=SL
  Bit Rotate3 : hdlsllib/Logic and Bit Operations/Bit Rotate  mode=Rotate Left  N=4
      settings: SourceProductName=Simulink  SourceProductBaseCode=SL
  Bit Rotate4 : hdlsllib/Logic and Bit Operations/Bit Rotate  mode=Rotate Left  N=5
      settings: SourceProductName=Simulink  SourceProductBaseCode=SL
  Bit Rotate5 : hdlsllib/Logic and Bit Operations/Bit Rotate  mode=Rotate Left  N=6
      settings: SourceProductName=Simulink  SourceProductBaseCode=SL
  Bit Rotate6 : hdlsllib/Logic and Bit Operations/Bit Rotate  mode=Rotate Left  N=7
      settings: SourceProductName=Simulink  SourceProductBaseCode=SL
  Bit Rotate7 : hdlsllib/Logic and Bit Operations/Bit Rotate  mode=Rotate Left  N=8
      settings: SourceProductName=Simulink  SourceProductBaseCode=SL
  Bit Rotate8 : hdlsllib/Logic and Bit Operations/Bit Rotate  mode=Rotate Left  N=9
      settings: SourceProductName=Simulink  SourceProductBaseCode=SL
  Bit Rotate9 : hdlsllib/Logic and Bit Operations/Bit Rotate  mode=Rotate Left  N=10
      settings: SourceProductName=Simulink  SourceProductBaseCode=SL
  Multiport Switch : MultiPortSwitch  DataPortOrder=Zero-based contiguous  Inputs=16  DiagnosticForDefault=Warning  zeroidx=on
  x_shifted : Outport
  wires:
  Bit Rotate14/1 -> Multiport Switch/17
  Bit Rotate13/1 -> Multiport Switch/16
  Bit Rotate12/1 -> Multiport Switch/15
  Bit Rotate11/1 -> Multiport Switch/14
  Bit Rotate10/1 -> Multiport Switch/13
  Bit Rotate9/1 -> Multiport Switch/12
  Bit Rotate8/1 -> Multiport Switch/11
  Bit Rotate7/1 -> Multiport Switch/10
  Bit Rotate6/1 -> Multiport Switch/9
  Bit Rotate5/1 -> Multiport Switch/8
  Bit Rotate4/1 -> Multiport Switch/7
  Bit Rotate3/1 -> Multiport Switch/6
  Bit Rotate2/1 -> Multiport Switch/5
  Bit Rotate1/1 -> Multiport Switch/4
  Bit Rotate/1 -> Multiport Switch/3
  x_in/1 -> Bit Rotate6/1, Bit Rotate3/1, Bit Rotate2/1, Bit Rotate1/1, Bit Rotate/1, Multiport Switch/2, Bit Rotate4/1, Bit Rotate5/1, Bit Rotate7/1, Bit Rotate8/1, Bit Rotate9/1, Bit Rotate10/1, Bit Rotate11/1, Bit Rotate14/1, Bit Rotate13/1, Bit Rotate12/1
  Multiport Switch/1 -> x_shifted/1
  NShifts/1 -> Multiport Switch/1

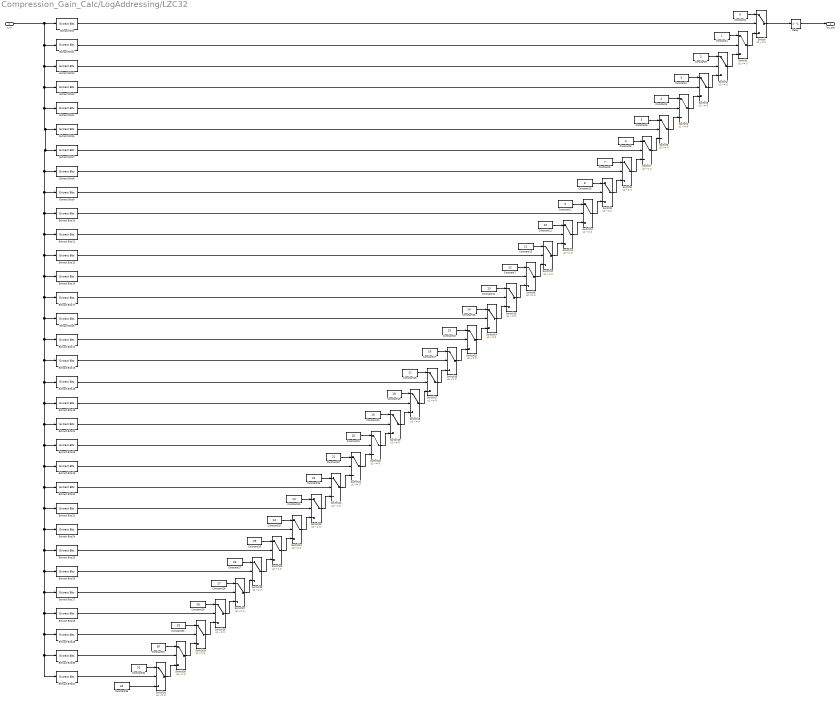
== system Compression_Gain_Calc/LogAddressing/LZC32 ==
  x_in : Inport
  Constant1 : Constant  OutDataTypeStr=fixdt(0,6,0)  SampleTime=Ts_system
  Constant10 : Constant  Value=8  OutDataTypeStr=fixdt(0,6,0)  SampleTime=Ts_system
  Constant11 : Constant  Value=9  OutDataTypeStr=fixdt(0,6,0)  SampleTime=Ts_system
  Constant12 : Constant  Value=10  OutDataTypeStr=fixdt(0,6,0)  SampleTime=Ts_system
  Constant13 : Constant  Value=11  OutDataTypeStr=fixdt(0,6,0)  SampleTime=Ts_system
  Constant14 : Constant  Value=13  OutDataTypeStr=fixdt(0,6,0)  SampleTime=Ts_system
  Constant15 : Constant  Value=14  OutDataTypeStr=fixdt(0,6,0)  SampleTime=Ts_system
  Constant16 : Constant  Value=15  OutDataTypeStr=fixdt(0,6,0)  SampleTime=Ts_system
  Constant17 : Constant  Value=16  OutDataTypeStr=fixdt(0,6,0)  SampleTime=Ts_system
  Constant18 : Constant  Value=17  OutDataTypeStr=fixdt(0,6,0)  SampleTime=Ts_system
  Constant19 : Constant  Value=18  OutDataTypeStr=fixdt(0,6,0)  SampleTime=Ts_system
  Constant2 : Constant  Value=0  OutDataTypeStr=fixdt(0,6,0)  SampleTime=Ts_system
  Constant20 : Constant  Value=19  OutDataTypeStr=fixdt(0,6,0)  SampleTime=Ts_system
  Constant21 : Constant  Value=20  OutDataTypeStr=fixdt(0,6,0)  SampleTime=Ts_system
  Constant22 : Constant  Value=21  OutDataTypeStr=fixdt(0,6,0)  SampleTime=Ts_system
  Constant23 : Constant  Value=22  OutDataTypeStr=fixdt(0,6,0)  SampleTime=Ts_system
  Constant24 : Constant  Value=23  OutDataTypeStr=fixdt(0,6,0)  SampleTime=Ts_system
  Constant25 : Constant  Value=24  OutDataTypeStr=fixdt(0,6,0)  SampleTime=Ts_system
  Constant26 : Constant  Value=25  OutDataTypeStr=fixdt(0,6,0)  SampleTime=Ts_system
  Constant27 : Constant  Value=26  OutDataTypeStr=fixdt(0,6,0)  SampleTime=Ts_system
  Constant28 : Constant  Value=27  OutDataTypeStr=fixdt(0,6,0)  SampleTime=Ts_system
  Constant29 : Constant  Value=28  OutDataTypeStr=fixdt(0,6,0)  SampleTime=Ts_system
  Constant3 : Constant  Value=2  OutDataTypeStr=fixdt(0,6,0)  SampleTime=Ts_system
  Constant30 : Constant  Value=29  OutDataTypeStr=fixdt(0,6,0)  SampleTime=Ts_system
  Constant31 : Constant  Value=30  OutDataTypeStr=fixdt(0,6,0)  SampleTime=Ts_system
  Constant32 : Constant  Value=31  OutDataTypeStr=fixdt(0,6,0)  SampleTime=Ts_system
  Constant33 : Constant  Value=32  OutDataTypeStr=fixdt(0,6,0)  SampleTime=Ts_system
  Constant4 : Constant  Value=3  OutDataTypeStr=fixdt(0,6,0)  SampleTime=Ts_system
  Constant5 : Constant  Value=4  OutDataTypeStr=fixdt(0,6,0)  SampleTime=Ts_system
  Constant6 : Constant  Value=5  OutDataTypeStr=fixdt(0,6,0)  SampleTime=Ts_system
  Constant7 : Constant  Value=12  OutDataTypeStr=fixdt(0,6,0)  SampleTime=Ts_system
  Constant8 : Constant  Value=6  OutDataTypeStr=fixdt(0,6,0)  SampleTime=Ts_system
  Constant9 : Constant  Value=7  OutDataTypeStr=fixdt(0,6,0)  SampleTime=Ts_system
  Delay : Delay  DelayLength=1  InitialCondition=3  SampleTime=Ts_system
  Extract Bits : simulink/Logic and Bit Operations/Extract Bits  bitsToExtract=Range of bits  numBits=8  bitIdxRange=[31 31]  outScalingMode=Treat bit field as an integer
      settings: SourceProductName=Simulink
  Extract Bits1 : simulink/Logic and Bit Operations/Extract Bits  bitsToExtract=Range of bits  numBits=8  bitIdxRange=[30 30]  outScalingMode=Treat bit field as an integer
      settings: SourceProductName=Simulink
  Extract Bits10 : simulink/Logic and Bit Operations/Extract Bits  bitsToExtract=Range of bits  numBits=8  bitIdxRange=[22 22]  outScalingMode=Treat bit field as an integer
      settings: SourceProductName=Simulink
  Extract Bits11 : simulink/Logic and Bit Operations/Extract Bits  bitsToExtract=Range of bits  numBits=8  bitIdxRange=[21 21]  outScalingMode=Treat bit field as an integer
      settings: SourceProductName=Simulink
  Extract Bits12 : simulink/Logic and Bit Operations/Extract Bits  bitsToExtract=Range of bits  numBits=8  bitIdxRange=[20 20]  outScalingMode=Treat bit field as an integer
      settings: SourceProductName=Simulink
  Extract Bits13 : simulink/Logic and Bit Operations/Extract Bits  bitsToExtract=Range of bits  numBits=8  bitIdxRange=[19 19]  outScalingMode=Treat bit field as an integer
      settings: SourceProductName=Simulink
  Extract Bits14 : simulink/Logic and Bit Operations/Extract Bits  bitsToExtract=Range of bits  numBits=8  bitIdxRange=[16 16]  outScalingMode=Treat bit field as an integer
      settings: SourceProductName=Simulink
  Extract Bits15 : simulink/Logic and Bit Operations/Extract Bits  bitsToExtract=Range of bits  numBits=8  bitIdxRange=[15 15]  outScalingMode=Treat bit field as an integer
      settings: SourceProductName=Simulink
  Extract Bits16 : simulink/Logic and Bit Operations/Extract Bits  bitsToExtract=Range of bits  numBits=8  bitIdxRange=[14 14]  outScalingMode=Treat bit field as an integer
      settings: SourceProductName=Simulink
  Extract Bits17 : simulink/Logic and Bit Operations/Extract Bits  bitsToExtract=Range of bits  numBits=8  bitIdxRange=[18 18]  outScalingMode=Treat bit field as an integer
      settings: SourceProductName=Simulink
  Extract Bits18 : simulink/Logic and Bit Operations/Extract Bits  bitsToExtract=Range of bits  numBits=8  bitIdxRange=[13 13]  outScalingMode=Treat bit field as an integer
      settings: SourceProductName=Simulink
  Extract Bits19 : simulink/Logic and Bit Operations/Extract Bits  bitsToExtract=Range of bits  numBits=8  bitIdxRange=[10 10]  outScalingMode=Treat bit field as an integer
      settings: SourceProductName=Simulink
  Extract Bits2 : simulink/Logic and Bit Operations/Extract Bits  bitsToExtract=Range of bits  numBits=8  bitIdxRange=[29 29]  outScalingMode=Treat bit field as an integer
      settings: SourceProductName=Simulink
  Extract Bits20 : simulink/Logic and Bit Operations/Extract Bits  bitsToExtract=Range of bits  numBits=8  bitIdxRange=[9 9]  outScalingMode=Treat bit field as an integer
      settings: SourceProductName=Simulink
  Extract Bits21 : simulink/Logic and Bit Operations/Extract Bits  bitsToExtract=Range of bits  numBits=8  bitIdxRange=[8 8]  outScalingMode=Treat bit field as an integer
      settings: SourceProductName=Simulink
  Extract Bits22 : simulink/Logic and Bit Operations/Extract Bits  bitsToExtract=Range of bits  numBits=8  bitIdxRange=[12 12]  outScalingMode=Treat bit field as an integer
      settings: SourceProductName=Simulink
  Extract Bits23 : simulink/Logic and Bit Operations/Extract Bits  bitsToExtract=Range of bits  numBits=8  bitIdxRange=[11 11]  outScalingMode=Treat bit field as an integer
      settings: SourceProductName=Simulink
  Extract Bits24 : simulink/Logic and Bit Operations/Extract Bits  bitsToExtract=Range of bits  numBits=8  bitIdxRange=[7 7]  outScalingMode=Treat bit field as an integer
      settings: SourceProductName=Simulink
  Extract Bits25 : simulink/Logic and Bit Operations/Extract Bits  bitsToExtract=Range of bits  numBits=8  bitIdxRange=[6 6]  outScalingMode=Treat bit field as an integer
      settings: SourceProductName=Simulink
  Extract Bits26 : simulink/Logic and Bit Operations/Extract Bits  bitsToExtract=Range of bits  numBits=8  bitIdxRange=[5 5]  outScalingMode=Treat bit field as an integer
      settings: SourceProductName=Simulink
  Extract Bits27 : simulink/Logic and Bit Operations/Extract Bits  bitsToExtract=Range of bits  numBits=8  bitIdxRange=[4 4]  outScalingMode=Treat bit field as an integer
      settings: SourceProductName=Simulink
  Extract Bits28 : simulink/Logic and Bit Operations/Extract Bits  bitsToExtract=Range of bits  numBits=8  bitIdxRange=[3 3]  outScalingMode=Treat bit field as an integer
      settings: SourceProductName=Simulink
  Extract Bits29 : simulink/Logic and Bit Operations/Extract Bits  bitsToExtract=Range of bits  numBits=8  bitIdxRange=[2 2]  outScalingMode=Treat bit field as an integer
      settings: SourceProductName=Simulink
  Extract Bits3 : simulink/Logic and Bit Operations/Extract Bits  bitsToExtract=Range of bits  numBits=8  bitIdxRange=[28 28]  outScalingMode=Treat bit field as an integer
      settings: SourceProductName=Simulink
  Extract Bits30 : simulink/Logic and Bit Operations/Extract Bits  bitsToExtract=Range of bits  numBits=8  bitIdxRange=[1 1]  outScalingMode=Treat bit field as an integer
      settings: SourceProductName=Simulink
  Extract Bits31 : simulink/Logic and Bit Operations/Extract Bits  bitsToExtract=Range of bits  numBits=8  bitIdxRange=[0 0]  outScalingMode=Treat bit field as an integer
      settings: SourceProductName=Simulink
  Extract Bits4 : simulink/Logic and Bit Operations/Extract Bits  bitsToExtract=Range of bits  numBits=8  bitIdxRange=[27 27]  outScalingMode=Treat bit field as an integer
      settings: SourceProductName=Simulink
  Extract Bits5 : simulink/Logic and Bit Operations/Extract Bits  bitsToExtract=Range of bits  numBits=8  bitIdxRange=[26 26]  outScalingMode=Treat bit field as an integer
      settings: SourceProductName=Simulink
  Extract Bits6 : simulink/Logic and Bit Operations/Extract Bits  bitsToExtract=Range of bits  numBits=8  bitIdxRange=[17 17]  outScalingMode=Treat bit field as an integer
      settings: SourceProductName=Simulink
  Extract Bits7 : simulink/Logic and Bit Operations/Extract Bits  bitsToExtract=Range of bits  numBits=8  bitIdxRange=[25 25]  outScalingMode=Treat bit field as an integer
      settings: SourceProductName=Simulink
  Extract Bits8 : simulink/Logic and Bit Operations/Extract Bits  bitsToExtract=Range of bits  numBits=8  bitIdxRange=[24 24]  outScalingMode=Treat bit field as an integer
      settings: SourceProductName=Simulink
  Extract Bits9 : simulink/Logic and Bit Operations/Extract Bits  bitsToExtract=Range of bits  numBits=8  bitIdxRange=[23 23]  outScalingMode=Treat bit field as an integer
      settings: SourceProductName=Simulink
  Switch{,1..31} (32 alike) : Switch  Criteria=u2 ~= 0
  lzc_out : Outport
  wires:
  x_in/1 -> Extract Bits31/1, Extract Bits30/1, Extract Bits29/1, Extract Bits28/1, Extract Bits27/1, Extract Bits26/1, Extract Bits25/1, Extract Bits24/1, Extract Bits21/1, Extract Bits20/1, Extract Bits19/1, Extract Bits23/1, Extract Bits22/1, Extract Bits18/1, Extract Bits16/1, Extract Bits15/1, Extract Bits14/1, Extract Bits6/1, Extract Bits17/1, Extract Bits13/1, Extract Bits12/1, Extract Bits11/1, Extract Bits10/1, Extract Bits9/1, Extract Bits8/1, Extract Bits7/1, Extract Bits5/1, Extract Bits4/1, Extract Bits3/1, Extract Bits2/1, Extract Bits1/1, Extract Bits/1
  Switch4/1 -> Switch3/3
  Extract Bits31/1 -> Switch31/2
  Constant28/1 -> Switch27/1
  Switch2/1 -> Switch1/3
  Extract Bits1/1 -> Switch1/2
  Switch6/1 -> Switch12/3
  Switch5/1 -> Switch4/3
  Constant14/1 -> Switch13/1
  Constant31/1 -> Switch30/1
  Extract Bits/1 -> Switch/2
  Constant33/1 -> Switch31/3
  Switch24/1 -> Switch23/3
  Switch14/1 -> Switch13/3
  Extract Bits27/1 -> Switch27/2
  Constant16/1 -> Switch15/1
  Extract Bits4/1 -> Switch4/2
  Constant3/1 -> Switch2/1
  Extract Bits30/1 -> Switch30/2
  Constant1/1 -> Switch1/1
  Extract Bits15/1 -> Switch16/2
  Switch3/1 -> Switch2/3
  Extract Bits19/1 -> Switch21/2
  Extract Bits2/1 -> Switch2/2
  Switch26/1 -> Switch25/3
  Switch18/1 -> Switch17/3
  Extract Bits21/1 -> Switch23/2
  Extract Bits28/1 -> Switch28/2
  Switch29/1 -> Switch28/3
  Switch20/1 -> Switch19/3
  Extract Bits14/1 -> Switch15/2
  Extract Bits23/1 -> Switch20/2
  Constant15/1 -> Switch14/1
  Extract Bits6/1 -> Switch14/2
  Constant17/1 -> Switch16/1
  Extract Bits5/1 -> Switch5/2
  Extract Bits18/1 -> Switch18/2
  Extract Bits20/1 -> Switch22/2
  Extract Bits26/1 -> Switch26/2
  Extract Bits22/1 -> Switch19/2
  Switch11/1 -> Switch10/3
  Extract Bits12/1 -> Switch12/2
  Extract Bits17/1 -> Switch13/2
  Extract Bits24/1 -> Switch24/2
  Switch28/1 -> Switch27/3
  Constant11/1 -> Switch10/1
  Constant8/1 -> Switch7/1
  Extract Bits25/1 -> Switch25/2
  Switch16/1 -> Switch15/3
  Extract Bits29/1 -> Switch29/2
  Switch9/1 -> Switch8/3
  Switch31/1 -> Switch30/3
  Switch19/1 -> Switch18/3
  Extract Bits9/1 -> Switch9/2
  Switch7/1 -> Switch5/3
  Extract Bits13/1 -> Switch6/2
  Extract Bits11/1 -> Switch11/2
  Constant18/1 -> Switch17/1
  Constant4/1 -> Switch3/1
  Extract Bits10/1 -> Switch10/2
  Extract Bits8/1 -> Switch8/2
  Extract Bits7/1 -> Switch7/2
  Constant2/1 -> Switch/1
  Constant22/1 -> Switch21/1
  Switch15/1 -> Switch14/3
  Switch30/1 -> Switch29/3
  Switch13/1 -> Switch6/3
  Switch17/1 -> Switch16/3
  Constant7/1 -> Switch6/1
  Constant30/1 -> Switch29/1
  Constant29/1 -> Switch28/1
  Switch27/1 -> Switch26/3
  Constant32/1 -> Switch31/1
  Constant26/1 -> Switch25/1
  Constant27/1 -> Switch26/1
  Switch25/1 -> Switch24/3
  Constant25/1 -> Switch24/1
  Constant10/1 -> Switch9/1
  Switch12/1 -> Switch11/3
  Switch8/1 -> Switch7/3
  Constant12/1 -> Switch11/1
  Switch21/1 -> Switch20/3
  Switch10/1 -> Switch9/3
  Constant13/1 -> Switch12/1
  Constant9/1 -> Switch8/1
  Constant23/1 -> Switch22/1
  Constant24/1 -> Switch23/1
  Switch22/1 -> Switch21/3
  Switch23/1 -> Switch22/3
  Constant20/1 -> Switch19/1
  Constant21/1 -> Switch20/1
  Constant19/1 -> Switch18/1
  Extract Bits16/1 -> Switch17/2
  Switch1/1 -> Switch/3
  Constant5/1 -> Switch4/1
  Constant6/1 -> Switch5/1
  Extract Bits3/1 -> Switch3/2
  Switch/1 -> Delay/1
  Delay/1 -> lzc_out/1

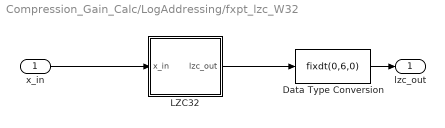
== system Compression_Gain_Calc/LogAddressing/fxpt_lzc_W32 ==
  x_in : Inport
  Data Type Conversion : DataTypeConversion  OutDataTypeStr=fixdt(0,6,0)
  LZC32 : Subsystem  TreatAsAtomicUnit=on
  lzc_out : Outport
  wires:
  LZC32/1(lzc_out) -> Data Type Conversion/1
  x_in/1 -> LZC32/1(x_in)
  Data Type Conversion/1 -> lzc_out/1
